simulink model "S_ET_PROP_V1"  (R2017a)
settings: Solver=FixedStepDiscrete  StartTime=0.0  StopTime=10.0  RelTol=1e-3
undefined symbols (not defined in the file or in its folder): Down, GPTRIP1SEL, GPTRIP2SEL, TZ1, TZ2, Up
libraries: c2802xlib x3, c2806xlib x2
settings Model: ExtModeTrigDuration=8  Creator=dricl  LastModifiedBy=dricl
settings OptimizationCC: DefaultUnderspecifiedDataType=single  PassReuseOutputArgsAs=Individual arguments  MaxStackSize=512
settings DebuggingCC: ParameterTunabilityLossMsg=error
settings HardwareCC: ProdBitPerChar=16  ProdBitPerInt=16  ProdBitPerPointer=32  ProdBitPerSizeT=32  ProdBitPerPtrDiffT=32  ProdLargestAtomicInteger=Integer  ProdLargestAtomicFloat=None  ProdWordSize=16  ProdLongLongMode=on  ProdHWDeviceType=Texas Instruments->C2000
settings SFSimCC: MATLABDynamicMemAlloc=off
settings RTWCC: SystemTargetFile=ert.tlc  HardwareBoard=TI Piccolo F2806x  TLCOptions=-aInlineSetEventsForThisBaseRateFcn=TLC_FALSE -aSuppressMultiTaskScheduler=TLC_FALSE -aRateBasedStepFcn=1  TemplateMakefile=ert_default_tmf  Description=Embedded Coder  Toolchain=Texas Instruments Code Composer Studio v5 (C2000)  CodeExecutionProfiling=on  CodeProfilingSaveOptions=AllData  CodeProfilingInstrumentation=on
settings CodeAppCC: ForceParamTrailComments=on  IgnoreCustomStorageClasses=off  OperatorAnnotations=on  SimulinkDataObjDesc=on  SFDataObjDesc=on  MATLABFcnDesc=on  InsertBlockDesc=on  MATLABSourceComments=on
settings ERTTargetCC: CodeReplacementLibrary=TI C28x  SupportVariableSizeSignals=on  MemSecPackage=tic2000demospkg  MemSecFuncExecute=code_ramfuncs

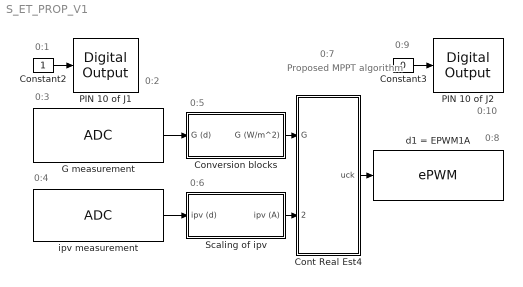
== system S_ET_PROP_V1 ==
  note: 0:1
  note: 0:2
  note: 0:3
  note: 0:4
  note: 0:5
  note: 0:6
  note: 0:7
  note: 0:8
  note: 0:9
  note: 0:10
  note: Proposed
      | MPPT algorithm
  Constant2 : Constant  Priority=1  SampleTime=0.0002
  Constant3 : Constant  Priority=9  Value=0  SampleTime=0.0002
  Cont Real Est4 : Subsystem  Priority=7
  Conversion blocks : Subsystem  Priority=5  TreatAsAtomicUnit=on
  G measurement : c2802xlib/ADC  Priority=3  ADCModule=1  samplingMode=Single sample mode  ADCResolution=12-bit (Single-ended input)  useSOC1=SOC1  useSOC2=SOC0_SOC1  SOCAcquisitionWindow=7  SOCTriggerSource=ePWM1_ADCSOCA  SOCInterruptTrigger=No ADCINT  Ts=0.0002  dType=uint16  postInterrupt=off  interruptSel=ADCINT1  ADCINTContinuous=on  endma=off  chdma=1  blkParamProc=C2000  conv1=ADCINA1  conv2=ADCINA0 and ADCINB0  conv1_Type4=ADCIN0  conv2_Type4=ADCIN0 and ADCIN1
      settings: SourceProductName=Embedded Coder Support Package for Texas Instruments C2000 Processors
  PIN 10 of J1 : c2806xlib/Digital Output  Priority=2  GPIO_Number=GPIO32~GPIO39  GPIO_Bit0=on  GPIO_BIT0_Toggle=off  GPIO_Bit1=off  GPIO_BIT1_Toggle=off  GPIO_Bit2=off  GPIO_BIT2_Toggle=off  GPIO_Bit3=off  GPIO_BIT3_Toggle=off  GPIO_Bit4=off  GPIO_BIT4_Toggle=off  GPIO_Bit5=off  GPIO_BIT5_Toggle=off  GPIO_Bit6=off  GPIO_BIT6_Toggle=off  GPIO_Bit7=off  GPIO_BIT7_Toggle=off
      settings: SourceProductName=Embedded Coder Support Package for Texas Instruments C2000 Processors  SourceProductBaseCode=TIC2000
  PIN 10 of J2 : c2806xlib/Digital Output  Priority=10  GPIO_Number=GPIO32~GPIO39  GPIO_Bit0=on  GPIO_BIT0_Toggle=off  GPIO_Bit1=off  GPIO_BIT1_Toggle=off  GPIO_Bit2=off  GPIO_BIT2_Toggle=off  GPIO_Bit3=off  GPIO_BIT3_Toggle=off  GPIO_Bit4=off  GPIO_BIT4_Toggle=off  GPIO_Bit5=off  GPIO_BIT5_Toggle=off  GPIO_Bit6=off  GPIO_BIT6_Toggle=off  GPIO_Bit7=off  GPIO_BIT7_Toggle=off
      settings: SourceProductName=Embedded Coder Support Package for Texas Instruments C2000 Processors  SourceProductBaseCode=TIC2000
  Scaling of ipv : Subsystem  Priority=6  TreatAsAtomicUnit=on
  d1 = EPWM1A : c2802xlib/ePWM  Priority=8  useModule=ePWM1  ePWMxLINKTBPRD=Not Linked  periodUnits=Clock cycles  timerSource=Specify via dialog  timerPeriod_clk=9000  timerPeriod_sec=0.0001  tbshadow=Counter equals to zero  countingMode=Up-Down  phaseActiveEnable=Disable  phaseDirection=Count down after sync  phaseActive=0  synchronizationEnable=off  dcaevt1Sync=off  dcbevt1Sync=off  synchronizationOption=Disable  clockPrescale=1  HSclockPrescale=1  enswap=off  ePWMxAStatus=on  ePWMxAactionLogic1=Do nothing  ePWMxAactionLogic2=Do nothing  ePWMxAactionLogic3=Clear  ePWMxAactionLogic4=Set  ePWMxAactionLogic5=Do nothing  ePWMxAactionLogic6=Do nothing  ePWMxALoadMode=Load on counter equals to zero (CTR=Zero)  ePWMxACSFenable=off  ePWMxACSFvalue=Forcing disable  ePWMxASFreload=Zero  ePWMxBStatus=off  ePWMxBactionLogic1=Set  ePWMxBactionLogic2=Clear  ePWMxBactionLogic3=Do nothing  ePWMxBactionLogic4=Do nothing  ePWMxBactionLogic5=Clear  ePWMxBactionLogic6=Set  ePWMxBLoadMode=Load on counter equals to zero (CTR=Zero)  ePWMxBCSFenable=off  ePWMxBCSFvalue=Forcing disable  ePWMxBSFreload=Zero  ePWNxBOutWay=off  ePWMxLINKCMPA=Not Linked  CMPAUnits=Clock cycles  CMPASource=Input port  CMPAValue_per=50  CMPAValue_clk=4500  enCMPAshadow=Counter equals to zero  ePWMxLINKCMPB=Not Linked  CMPBUnits=Clock cycles  CMPBSource=Specify via dialog  CMPBValue_per=50  CMPBValue_clk=4500  enCMPBshadow=Counter equals to zero  ePWMxLINKCMPC=Not Linked  CMPCUnits=Clock cycles  CMPCSource=Specify via dialog  CMPCValue_per=50  CMPCValue_clk=32000  enCMPCshadow=Counter equals to zero  ePWMxLINKCMPD=Not Linked  CMPDUnits=Clock cycles  CMPDSource=Specify via dialog  CMPDValue_per=50  CMPDValue_clk=32000  enCMPDshadow=Counter equals to zero  enableDBePWMxA=on  enableDBePWMxB=on  enhalfcycle=off  DBpolarity=Active high complementary (AHC)  DBedgeDelay=Positive  DBSource_ePWMxA=ePWMxA  DBSource_ePWMxB=ePWMxA  DBperiodSource=Specify via dialog  REDperiod=50  FEDperiod=50  adcstartModuleA=on  adcrequestEventA=First event  adcstartEventA=Counter equals to period (CTR=PRD)  adcstartEventA_type2=Digital Compare Module A Event 1 start of conversion (DCAEVT1.soc)  adcstartModuleB=off  adcrequestEventB=First event  adcstartEventB=Counter equals to zero (CTR=Zero)  adcstartEventB_type2=Counter equals to zero (CTR=Zero)  intEn=off  intPrd=First event  intSel=Counter equals to zero (CTR=Zero)  intSel_type2=Counter equals to zero (CTR=Zero)  hrpe=off  enHRPWM=off  HRPWM_LoadMode=Counter equals to period (CTR=PRD)  HRPWM_CTLMode=Duty or Period control mode  HRPWM_EDGMode=Both edge  hrpeb=off  enHRPWMB=off  HRPWM_LoadModeB=Counter equals to zero (CTR=ZERO)  HRPWM_CTLModeB=Duty or Period control mode  HRPWM_EDGModeB=Both edge  enSFO=on  enautoconv=on  chopperEnable=off  chopperFrequency=1  chopperFirstwidth=1  chopperDuty=12.5%  tripZonesource=Specify via dialog  tzselOSHT1=off  tzselOSHT2=off  tzselOSHT3=off  tzselOSHDCAEV1=off  tzselOSHDCBEV1=off  tzselCBC1=off  tzselCBC2=off  tzselCBC3=off  tzselCBCDCAEV2=off  tzselCBCDCBEV2=off  tzselOSHT4=off  tzselOSHT5=off  tzselOSHT6=off  tzselCBC4=off  tzselCBC5=off  tzselCBC6=off  enTzOstIntr=off  enTzCbcIntr=off  enTzDCAEVT1Intr=off  enTzDCAEVT2Intr=off  enTzDCBEVT1Intr=off  enTzDCBEVT2Intr=off  ePWMxAforced=No action  ePWMxBforced=No action  DCAEVT1forced=No action  DCBEVT1forced=No action  DCAEVT2forced=No action  DCBEVT2forced=No action  dcah=Trip Zone 1 input (TZ1)  dcal=Trip Zone 2 input (TZ2)  dcbh=Trip Zone 1 input (TZ1)  dcbl=Trip Zone 2 input (TZ2)  dcah_type2=GPTRIP1SEL/(TZ1)  dcal_type2=GPTRIP2SEL/(TZ2)  dcbh_type2=GPTRIP1SEL/(TZ1)  dcbl_type2=GPTRIP2SEL/(TZ2)  gendcaevt1=Event disabled  gendcaevt2=Event disabled  gendcbevt1=Event disabled  gendcbevt2=Event disabled  dcaevt1src=DCAEVT1 with sync  dcaevt2src=DCAEVT2 with sync  dcbevt1src=DCBEVT1 with sync  dcbevt2src=DCBEVT2 with sync  pulsesel=Counter equals to zero (CTR=Zero)  blankinv=off  blankoffset=0  blankwidth=0  evsrcsel=Filtered version of DCAEVT1 (DCAEVT1FILT)  encape=off  PwmType=C2000
      settings: SourceProductName=Embedded Coder Support Package for Texas Instruments C2000 Processors
  ipv measurement : c2802xlib/ADC  Priority=4  ADCModule=1  samplingMode=Single sample mode  ADCResolution=12-bit (Single-ended input)  useSOC1=SOC2  useSOC2=SOC0_SOC1  SOCAcquisitionWindow=7  SOCTriggerSource=ePWM1_ADCSOCA  SOCInterruptTrigger=No ADCINT  Ts=0.0002  dType=uint16  postInterrupt=off  interruptSel=ADCINT1  ADCINTContinuous=on  endma=off  chdma=1  blkParamProc=C2000  conv1=ADCINA0  conv2=ADCINA0 and ADCINB0  conv1_Type4=ADCIN0  conv2_Type4=ADCIN0 and ADCIN1
      settings: SourceProductName=Embedded Coder Support Package for Texas Instruments C2000 Processors
  wires:
  Scaling of ipv/1(ipv (A)) -> Cont Real Est4/2(x1 = ipv)
  ipv measurement/1 -> Scaling of ipv/1(ipv (d))
  Conversion blocks/1(G (W/m^2)) -> Cont Real Est4/1(G)
  G measurement/1 -> Conversion blocks/1(G (d))
  Constant2/1 -> PIN 10 of J1/1
  Constant3/1 -> PIN 10 of J2/1
  Cont Real Est4/1(uck) -> d1 = EPWM1A/1

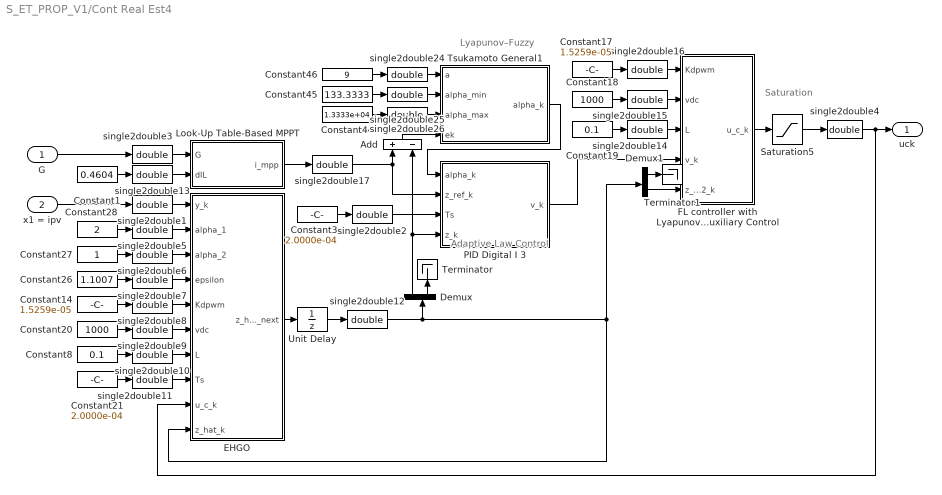
== system S_ET_PROP_V1/Cont Real Est4 ==
  note: Saturation
  note: Adaptive Law Control
  note: Lyapunov–Fuzzy
  G : Inport
  x1 = ipv : Inport  Port=2
  Add : Sum  Inputs=+-
  Constant1 : Constant  Value=0.4604  SampleTime=2.0000e-04
  Constant14 : Constant  Value=1.5259e-05  SampleTime=2.0000e-04
  Constant17 : Constant  Value=1.5259e-05  SampleTime=2.0000e-04
  Constant18 : Constant  Value=1000  SampleTime=2.0000e-04
  Constant19 : Constant  Value=0.1  SampleTime=2.0000e-04
  Constant20 : Constant  Value=1000  SampleTime=2.0000e-04
  Constant21 : Constant  Value=2.0000e-04  SampleTime=2.0000e-04
  Constant26 : Constant  Value=1.1007  SampleTime=2.0000e-04
  Constant27 : Constant  SampleTime=2.0000e-04
  Constant28 : Constant  Value=2  SampleTime=2.0000e-04
  Constant3 : Constant  Value=2.0000e-04  SampleTime=2.0000e-04
  Constant44 : Constant  Value=1.3333e+04  SampleTime=2.0000e-04
  Constant45 : Constant  Value=133.3333  SampleTime=2.0000e-04
  Constant46 : Constant  Value=9  SampleTime=2.0000e-04
  Constant8 : Constant  Value=0.1  SampleTime=2.0000e-04
  Demux : Demux  Outputs=2
  Demux1 : Demux  Outputs=2
  EHGO : MATLAB Function  TreatAsAtomicUnit=on
  FL controller with Lyapunov–Fuzzy Adaptive Auxiliary Control : MATLAB Function  TreatAsAtomicUnit=on
  Look-Up Table-Based MPPT : MATLAB Function  TreatAsAtomicUnit=on
  PID Digital I 3 : MATLAB Function  TreatAsAtomicUnit=on
  Saturation5 : Saturate  UpperLimit=9000*0.98  LowerLimit=9000*0.05
  Terminator : Terminator
  Terminator1 : Terminator
  Tsukamoto General1 : MATLAB Function  TreatAsAtomicUnit=on
  Unit Delay : UnitDelay  SampleTime=2.0000e-04
  single2double{1..17,24..26} (20 alike) : DataTypeConversion  OutDataTypeStr=double
  uck : Outport
  wires:
  x1 = ipv/1 -> single2double1/1
  FL controller with Lyapunov–Fuzzy Adaptive Auxiliary Control/1(u_c_k) -> Saturation5/1
  single2double1/1 -> EHGO/1(y_k)
  Saturation5/1 -> single2double4/1
  single2double4/1 -> EHGO/9(u_c_k), uck/1
  Constant28/1 -> single2double5/1
  single2double5/1 -> EHGO/2(alpha_1)
  Constant27/1 -> single2double6/1
  single2double6/1 -> EHGO/3(alpha_2)
  Constant26/1 -> single2double7/1
  single2double7/1 -> EHGO/4(epsilon)
  Constant14/1 -> single2double8/1
  single2double8/1 -> EHGO/5(Kdpwm)
  Constant20/1 -> single2double9/1
  single2double9/1 -> EHGO/6(vdc)
  Constant8/1 -> single2double10/1
  single2double10/1 -> EHGO/7(L)
  Constant21/1 -> single2double11/1
  single2double11/1 -> EHGO/8(Ts)
  Unit Delay/1 -> single2double12/1
  single2double12/1 -> Demux/1, EHGO/10(z_hat_k), Demux1/1
  Constant19/1 -> single2double14/1
  Constant18/1 -> single2double15/1
  Constant17/1 -> single2double16/1
  single2double16/1 -> FL controller with Lyapunov–Fuzzy Adaptive Auxiliary Control/1(Kdpwm)
  single2double15/1 -> FL controller with Lyapunov–Fuzzy Adaptive Auxiliary Control/2(vdc)
  single2double14/1 -> FL controller with Lyapunov–Fuzzy Adaptive Auxiliary Control/3(L)
  G/1 -> single2double3/1
  EHGO/1(z_hat_next) -> Unit Delay/1
  Constant3/1 -> single2double2/1
  single2double2/1 -> PID Digital I 3/3(Ts)
  Constant46/1 -> single2double24/1
  single2double25/1 -> Tsukamoto General1/2(alpha_min)
  Constant44/1 -> single2double26/1
  single2double26/1 -> Tsukamoto General1/3(alpha_max)
  single2double24/1 -> Tsukamoto General1/1(a)
  Constant45/1 -> single2double25/1
  Add/1 -> Tsukamoto General1/4(ek)
  Demux/2 -> Terminator/1
  Demux/1 -> PID Digital I 3/4(z_k), Add/2
  Tsukamoto General1/1(alpha_k) -> PID Digital I 3/1(alpha_k)
  single2double3/1 -> Look-Up Table-Based MPPT/1(G)
  Constant1/1 -> single2double13/1
  single2double13/1 -> Look-Up Table-Based MPPT/2(dIL)
  Demux1/2 -> FL controller with Lyapunov–Fuzzy Adaptive Auxiliary Control/5(z_hat_2_k)
  Demux1/1 -> Terminator1/1
  PID Digital I 3/1(v_k) -> FL controller with Lyapunov–Fuzzy Adaptive Auxiliary Control/4(v_k)
  single2double17/1 -> PID Digital I 3/2(z_ref_k), Add/1
  Look-Up Table-Based MPPT/1(i_mpp) -> single2double17/1

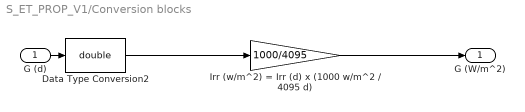
== system S_ET_PROP_V1/Conversion blocks ==
  G (d) : Inport
  Data Type Conversion2 : DataTypeConversion  OutDataTypeStr=double
  Irr (w/m^2) = Irr (d) x (1000 w/m^2 / 4095 d) : Gain  Gain=1000/4095
  G (W/m^2) : Outport
  wires:
  G (d)/1 -> Data Type Conversion2/1
  Data Type Conversion2/1 -> Irr (w/m^2) = Irr (d) x (1000 w/m^2 / 4095 d)/1
  Irr (w/m^2) = Irr (d) x (1000 w/m^2 / 4095 d)/1 -> G (W/m^2)/1

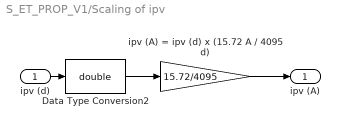
== system S_ET_PROP_V1/Scaling of ipv ==
  ipv (d) : Inport
  Data Type Conversion2 : DataTypeConversion  OutDataTypeStr=double
  ipv (A) = ipv (d) x (15.72 A / 4095 d) : Gain  Gain=15.72/4095
  ipv (A) : Outport
  wires:
  ipv (d)/1 -> Data Type Conversion2/1
  Data Type Conversion2/1 -> ipv (A) = ipv (d) x (15.72 A / 4095 d)/1
  ipv (A) = ipv (d) x (15.72 A / 4095 d)/1 -> ipv (A)/1

== matlab function S_ET_PROP_V1/Cont Real Est4/EHGO ==
  data: y_k input; alpha_1 input; alpha_2 input; epsilon input; Kdpwm input; vdc input; L input; Ts input; u_c_k input; z_hat_k input; z_hat_next output
function z_hat_next = fcn(y_k, alpha_1, alpha_2, epsilon, ...
                          Kdpwm, vdc, L, Ts, u_c_k, z_hat_k)
% Discrete-time extended high-gain observer (EHGO).
%
% Inputs:
%   y_k       : measured output y[k]
%   alpha_1   : first EHGO coefficient
%   alpha_2   : second EHGO coefficient
%   epsilon   : high-gain observer tuning parameter
%   Kdpwm     : DPWM gain
%   vdc       : dc-bus voltage
%   L         : Boost-converter inductance
%   Ts        : sampling period
%   u_c_k     : converter control input u_c[k]
%   z_hat_k   : current EHGO state estimates
%
% Output:
%   z_hat_next : EHGO state estimates at k+1

z_hat_next = zeros(2,1);

% Output-estimation error
e_obs_k = y_k - z_hat_k(1);

% EHGO state update
z_hat_next(1) = z_hat_k(1) + Ts * ( ...
    z_hat_k(2) + ...
    ((Kdpwm/L)*vdc)*u_c_k + ...
    (alpha_1/(epsilon*Ts))*e_obs_k );

z_hat_next(2) = z_hat_k(2) + Ts * ( ...
    (alpha_2/(epsilon^2*Ts^2))*e_obs_k );

end

== matlab function S_ET_PROP_V1/Cont Real Est4/FL controller with Lyapunov–Fuzzy Adaptive Auxiliary Control ==
  data: Kdpwm input; vdc input; L input; v_k input; u_c_k output; z_hat_2_k input
function u_c_k = fcn(Kdpwm, vdc, L, v_k, z_hat_2_k)
% Feedback-linearizing control law using the EHGO estimate.
%
% Inputs:
%   Kdpwm       : DPWM gain
%   vdc         : dc-bus voltage
%   L           : Boost-converter inductance
%   v_k         : LFA auxiliary control v[k]
%   z_hat_2_k   : second EHGO state estimate
%
% Output:
%   u_c_k       : converter control input u_c[k]

u_c_k = (L/(Kdpwm*vdc)) * ...
        (-z_hat_2_k + v_k);

end

== matlab function S_ET_PROP_V1/Cont Real Est4/Look-Up Table-Based MPPT ==
  data: G input; i_mpp output; dIL input
function i_mpp = fcn(G, dIL)
% MPP current reference generation using a G-to-Impp lookup table.
%
% G       : irradiance input
% dIL     : peak-to-peak inductor-current ripple compensation
%
% Output:
% i_mpp   : compensated MPP current reference
%
% The lookup table covers G = 50...1200 W/m^2 with a 10 W/m^2 step.
% Linear interpolation is used within the table and extrapolation is
% applied outside the tabulated irradiance range.

persistent G_tab Impp_tab

if isempty(G_tab)

    G_tab = single(50:10:1200);

    Impp_tab = coder.const(double([ ...
    0.79 0.95 1.10 1.26 1.42 1.58 1.74 1.89 2.05 2.21 ...
    2.36 2.53 2.68 2.84 3.00 3.15 3.31 3.47 3.63 3.78 ...
    3.95 4.10 4.26 4.41 4.58 4.73 4.89 5.05 5.21 5.36 ...
    5.52 5.68 5.84 5.99 6.15 6.31 6.46 6.62 6.78 6.94 ...
    7.09 7.25 7.41 7.57 7.72 7.88 8.04 8.20 8.36 8.51 ...
    8.67 8.83 8.98 9.13 9.29 9.45 9.61 9.76 9.92 10.08 ...
    10.24 10.39 10.55 10.71 10.86 11.02 11.18 11.33 11.49 11.64 ...
    11.80 11.96 12.11 12.28 12.44 12.60 12.75 12.90 13.06 13.21 ...
    13.37 13.52 13.68 13.85 14.01 14.16 14.31 14.47 14.62 14.77 ...
    14.92 15.10 15.25 15.41 15.56 15.71 15.86 16.04 16.19 16.34 ...
    16.49 16.64 16.80 16.96 17.12 17.27 17.42 17.57 17.75 17.90 ...
    18.05 18.20 18.35 18.53 18.68 18.83
    ]));

end

% Nominal MPP-current interpolation
I_mpp_nom = interp1(G_tab, Impp_tab, G, 'linear', 'extrap');

% Inductor-current ripple compensation
i_mpp = I_mpp_nom - dIL;

% Prevent negative current-reference values
i_mpp = max(i_mpp, 0);

end

== matlab function S_ET_PROP_V1/Cont Real Est4/PID Digital I 3 ==
  data: alpha_k input; z_ref_k input; Ts input; v_k output; z_k input
function v_k = fcn(alpha_k, z_ref_k, Ts, z_k)
% LFA auxiliary control implementation.
%
% The decay rate alpha[k], provided by the two-rule Tsukamoto fuzzy
% inference system, determines the discrete-time contraction factor
% lambda[k]. The adaptive gains K[k] and L[k] are then computed to
% generate the auxiliary control v[k].
%
% Inputs:
%   alpha_k : Decay rate alpha[k] provided by the fuzzy inference system
%   z_ref_k : Tracking reference z_ref[k] = i_mpp[k]
%   Ts      : Sampling period
%   z_k     : Feedback-linearized state z[k]
%
% Output:
%   v_k     : Auxiliary control v[k]

% Numerical protection
alpha_k = max(alpha_k, eps);

% Contraction factor - equation (35)
lambda_k = exp(-alpha_k * Ts);

% Adaptive auxiliary-control gains - equation (34)
K_k = (1 - lambda_k) / Ts;
L_k = (1 - lambda_k) / Ts;

% LFA auxiliary control law - equation (34)
v_k = -K_k * z_k + L_k * z_ref_k;

end

== matlab function S_ET_PROP_V1/Cont Real Est4/Tsukamoto General1 ==
  data: a input; alpha_min input; alpha_max input; ek input; alpha_k output
function alpha_k = fcn(a, alpha_min, alpha_max, ek)
% General two-rule Tsukamoto implementation with w1 = exp(...)
%
% ek         : tracking error (scalar or vector)
% a          : Gaussian width parameter for mu_A1(|ek|)
% alpha_min  : lower bound of the physical decay-rate interval
% alpha_max  : upper bound of the physical decay-rate interval
%
% Output:
% alpha_k    : decay rate alpha[k] in [alpha_min, alpha_max]

% Numerical protection
a = max(a, eps);

% Width of the physical decay-rate interval
Delta_alpha = alpha_max - alpha_min;

% Centered output universe
alpha_c_min = -Delta_alpha/2;
alpha_c_max =  Delta_alpha/2;

% Input fuzzification based on the tracking-error magnitude
e_abs = abs(ek);

w1 = exp(-(e_abs.^2)/(2*a^2));   % mu_A1(|ek|): small tracking error
w2 = 1 - w1;                     % mu_A2(|ek|): large tracking error

% Tsukamoto inversion for alpha_c in
% [alpha_c_min, alpha_c_max]
z1 = alpha_c_max - w1.*Delta_alpha;  % R1: A1 -> B2 (decreasing)
z2 = alpha_c_min + w2.*Delta_alpha;  % R2: A2 -> B1 (increasing)

% Normalized weighted aggregation in the centered universe
den = w1 + w2;
den(den < eps) = eps;

alpha_c = ...
    (w1.*z1 + w2.*z2) ./ den;

% Translation to the physical decay-rate interval
alpha_k = ...
    alpha_c + ...
    (alpha_min + alpha_max)/2;

% Optional numerical saturation
alpha_k = ...
    min(max(alpha_k, alpha_min), alpha_max);

end
